simulink model "model"  (R2015b)
settings: Solver=FixedStepAuto  SolverMode=SingleTasking  StartTime=0.0  StopTime=60  FixedStep=0.1  RelTol=1e-3  AbsTol=1e-6
settings Model: Creator=1  LastModifiedBy=Administrator
settings DataIOCC: LimitDataPoints=off  SaveFormat=Array  SignalLoggingSaveFormat=ModelDataLogs  SignalLoggingName=sigsOut
settings OptimizationCC: BooleanDataType=off  DefaultParameterBehavior=Inlined  EnhancedBackFolding=on  OptimizeModelRefInitCode=on  LifeSpan=1
settings DebuggingCC: SaveWithParameterizedLinksMsg=none  UnderspecifiedInitializationDetection=Classic  MergeDetectMultiDrivingBlocksExec=none  SignalResolutionControl=TryResolveAllWithWarning  MultiTaskDSMMsg=warning  MultiTaskCondExecSysMsg=none  ParameterTunabilityLossMsg=error  AllowSymbolicDim=on  SFUnexpectedBacktrackingDiag=error  SFNoUnconditionalDefaultTransitionDiag=error
settings HardwareCC: TargetBitPerPointer=64  TargetLongLongMode=on  TargetIntDivRoundTo=Zero  TargetEndianess=LittleEndian  TargetWordSize=64  TargetHWDeviceType=MATLAB Host  ProdEqTarget=off
settings RTWCC: SystemTargetFile=ert.tlc  GenCodeOnly=on  TemplateMakefile=ert_default_tmf  Description=Embedded Coder  GenerateReport=on  IncludeHyperlinkInReport=on  LaunchReport=on
settings CodeAppCC: ForceParamTrailComments=on  IgnoreCustomStorageClasses=off  OperatorAnnotations=on
settings ERTTargetCC: GenerateSampleERTMain=on  SupportContinuousTime=on  InlinedParameterPlacement=NonHierarchical  ERTCustomFileTemplate=example_file_process.tlc
settings ConfigComp: CovModelRefEnable=Off

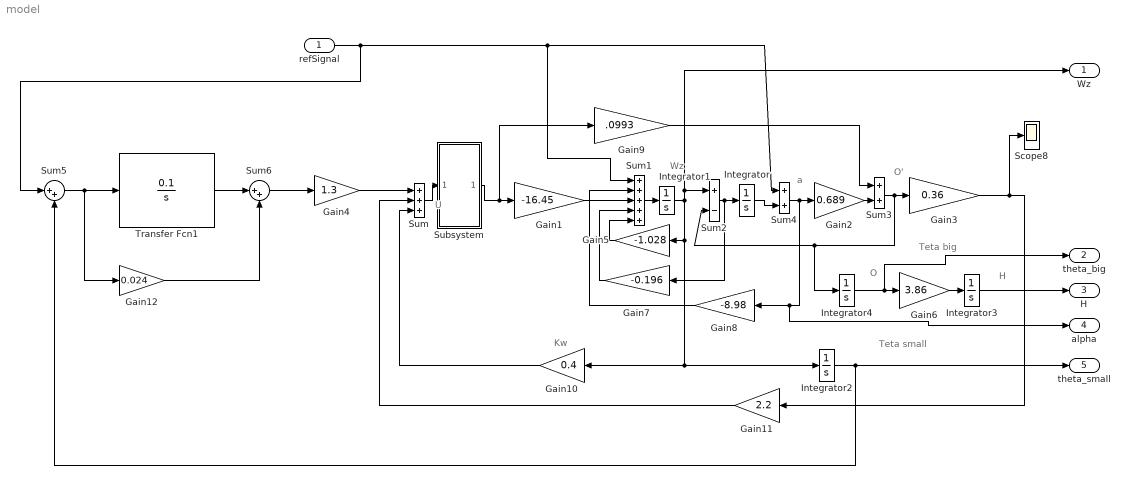
== system model ==
  note: U
  note: Wz
  note: Kw
  note: O'
  note: a
  note: Teta small
  note: O
  note: H
  note: Teta big
  refSignal : Inport
  Gain1 : Gain  Gain=-16.45  SaturateOnIntegerOverflow=on  OutDataTypeStr=Inherit: Same as input  ParamDataTypeStr=Inherit: Same as input
  Gain10 : Gain  Gain=0.4  SaturateOnIntegerOverflow=on  OutDataTypeStr=Inherit: Same as input  ParamDataTypeStr=Inherit: Same as input
  Gain11 : Gain  Gain=2.2  SaturateOnIntegerOverflow=on  OutDataTypeStr=Inherit: Same as input  ParamDataTypeStr=Inherit: Same as input
  Gain12 : Gain  Gain=0.024  SaturateOnIntegerOverflow=on  OutDataTypeStr=Inherit: Same as input  ParamDataTypeStr=Inherit: Same as input
  Gain2 : Gain  Gain=0.689  SaturateOnIntegerOverflow=on  OutDataTypeStr=Inherit: Same as input  ParamDataTypeStr=Inherit: Same as input
  Gain3 : Gain  Gain=0.36  SaturateOnIntegerOverflow=on  OutDataTypeStr=Inherit: Same as input  ParamDataTypeStr=Inherit: Same as input
  Gain4 : Gain  Gain=1.3  SaturateOnIntegerOverflow=on  OutDataTypeStr=Inherit: Same as input  ParamDataTypeStr=Inherit: Same as input
  Gain5 : Gain  Gain=-1.028  SaturateOnIntegerOverflow=on  OutDataTypeStr=Inherit: Same as input  ParamDataTypeStr=Inherit: Same as input
  Gain6 : Gain  Gain=3.86  SaturateOnIntegerOverflow=on  OutDataTypeStr=Inherit: Same as input  ParamDataTypeStr=Inherit: Same as input
  Gain7 : Gain  Gain=-0.196  SaturateOnIntegerOverflow=on  OutDataTypeStr=Inherit: Same as input  ParamDataTypeStr=Inherit: Same as input
  Gain8 : Gain  Gain=-8.98  SaturateOnIntegerOverflow=on  OutDataTypeStr=Inherit: Same as input  ParamDataTypeStr=Inherit: Same as input
  Gain9 : Gain  Gain=.0993  SaturateOnIntegerOverflow=on  OutDataTypeStr=Inherit: Same as input  ParamDataTypeStr=Inherit: Same as input
  Integrator{,1..4} (5 alike) : Integrator
  Scope8 : Scope
  Subsystem : Subsystem
  Sum : Sum  Inputs=+++  SaturateOnIntegerOverflow=on  InputSameDT=on  OutDataTypeStr=Inherit: Same as first input
  Sum1 : Sum  Inputs=+++++  SaturateOnIntegerOverflow=on  InputSameDT=on  OutDataTypeStr=Inherit: Same as first input
  Sum2 : Sum  Inputs=+-  SaturateOnIntegerOverflow=on  InputSameDT=on  OutDataTypeStr=Inherit: Same as first input
  Sum3 : Sum  SaturateOnIntegerOverflow=on  InputSameDT=on  OutDataTypeStr=Inherit: Same as first input
  Sum4 : Sum  SaturateOnIntegerOverflow=on  InputSameDT=on  OutDataTypeStr=Inherit: Same as first input
  Sum5 : Sum  Inputs=|++  SaturateOnIntegerOverflow=on
  Sum6 : Sum  Inputs=|++  SaturateOnIntegerOverflow=on
  Transfer Fcn1 : TransferFcn  Numerator=[0.1]  Denominator=[1 0]
  Wz : Outport
  theta_big : Outport  Port=2
  H : Outport  Port=3
  alpha : Outport  Port=4
  "theta_small " : Outport  Port=5
  wires:
  Sum2/1 -> Integrator/1, Gain7/1
  Integrator1/1 -> Gain5/1, Integrator2/1, Gain10/1, Wz/1, Sum2/1
  Gain9/1 -> Sum3/1
  Gain2/1 -> Sum3/2
  Sum3/1 -> Sum2/2, Integrator4/1, Gain3/1
  Sum1/1 -> Integrator1/1
  Gain10/1 -> Sum/3
  Gain11/1 -> Sum/2
  Gain3/1 -> Scope8/1, Gain11/1
  Gain5/1 -> Sum1/5
  Gain1/1 -> Sum1/2
  Gain8/1 -> Sum1/3
  Sum4/1 -> Gain2/1, alpha/1, Gain8/1
  Integrator/1 -> Sum4/2
  Integrator2/1 -> "theta_small "/1, Sum5/2
  Integrator4/1 -> theta_big/1, Gain6/1
  Gain6/1 -> Integrator3/1
  Integrator3/1 -> H/1
  Gain7/1 -> Sum1/4
  Sum/1 -> Subsystem/1(In1)
  Subsystem/1(Out1) -> Gain1/1, Gain9/1
  Sum6/1 -> Gain4/1
  refSignal/1 -> Sum5/1, Sum4/1, Sum1/1
  Gain4/1 -> Sum/1
  Sum5/1 -> Gain12/1, Transfer Fcn1/1
  Transfer Fcn1/1 -> Sum6/1
  Gain12/1 -> Sum6/2

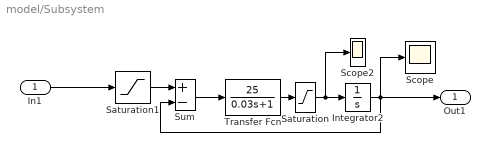
== system model/Subsystem ==
  In1 : Inport
  Integrator2 : Integrator  LimitOutput=on  UpperSaturationLimit=20  LowerSaturationLimit=-25
  Saturation : Saturate  UpperLimit=25  LowerLimit=-25
  Saturation1 : Saturate  UpperLimit=20  LowerLimit=-25
  Scope : Scope
  Scope2 : Scope
  Sum : Sum  Inputs=+-  SaturateOnIntegerOverflow=on  InputSameDT=on  OutDataTypeStr=Inherit: Same as first input
  Transfer Fcn : TransferFcn  Numerator=[25]  Denominator=[0.03 1]
  Out1 : Outport  InitialOutput=0
  wires:
  Transfer Fcn/1 -> Saturation/1
  Sum/1 -> Transfer Fcn/1
  Integrator2/1 -> Sum/2, Scope/1, Out1/1
  Saturation/1 -> Integrator2/1, Scope2/1
  Saturation1/1 -> Sum/1
  In1/1 -> Saturation1/1
